simulink model "warplab_mimo_4x4"  (Simulink 6.5)
settings: Solver=ode45  StartTime=0.0  StopTime=20000  RelTol=1e-3
undefined symbols (not defined in the file): gcbh, xlBlockLoadCallback
libraries: xbsIndex_r4 x188
(part 1 of 17)
settings Model: Creator=Melissa.Duarte  LastModifiedBy=melissa.duarte
settings DebuggingCC: MultiTaskDSMMsg=warning  MultiTaskCondExecSysMsg=none
settings RTWCC: IncludeERTFirstTime=on

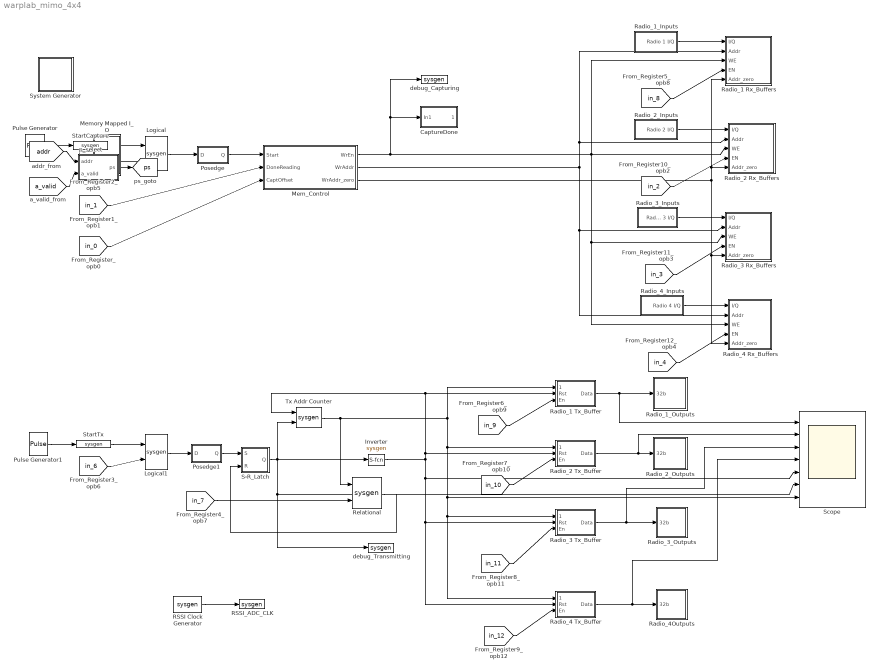
== system warplab_mimo_4x4 ==
  " System Generator" : Subsystem  Tag=genX  mask(Xilinx System Generator Block){infoedit=System Generator, xilinxfamily=virtex2p, part=xc2vp70, speed=-6, package=ff1517, synthesis_tool_sgadvanced=, synthesis_tool=XST, directory=./OPB_Export, testbench_sgadvanced=, testbench=off, simulink_period=1, sysclk_period=10, incr_netlist_sgadvanced=, incr_netlist=off, trim_vbits_sgadvanced=, trim_vbits=Everywhere in SubSystem, dbl_ovrd_sgadvanced=, dbl_ovrd=According to Block Masks, core_generation_sgadvanced=, core_generation=According to Block Masks, run_coregen_sgadvanced=, run_coregen=off, deprecated_control_sgadvanced=, deprecated_control=off, eval_field=0, has_advanced_control=0, sggui_pos=-1,-1,-1,-1, block_type=sysgen, block_version=8.2, sg_icon_stat=51,50,-1,-1,red,beige,0,07734, sg_mask_display=|, sg_list_contents=, sg_blockgui_xml=|}
      mask sg_mask_display=|
      | fprintf('','COMMENT: begin icon graphics');
      | patch([0 51 51 0 ],[0 0 50 50 ],[0.93 0.92 0.86]);
      | patch([12 4 16 4 12 25 29 33 47 36 25 17 29 17 25 36 47 33 29 25 12 ],[5 13 25 37 45 45 41 45 45 34 45 37 25 13 5 16 5 5 9 5 5 ],[0.6 0.2 0.25]);
      | plot([0 0 51 51 0 ],[0 50 50 0 0 ]);
      | fprintf('','COMMENT: end icon graphics');
      | fprintf('','COMMENT: begin icon text');
      | fprintf('','COMMENT: end icon text');
      mask sg_blockgui_xml=|
      | <!--  *  Copyright (c) 2005, Xilinx, Inc.  All Rights Reserved.            --><!--  *  Reproduction or reuse, in any form, without the explicit written  --><!--  *  consent of Xilinx, Inc., is strictly prohibited.                  --><sysgenblock has_userdata="true" tag="genX" block_type="sysgen" simulinkname=" System Generator" >
      |  <icon width="51" bg_color="beige" height="50" caption_format="System\nGenerator" wmark_color="red" />
      |  <callbacks DeleteFcn="xlSysgenGUI('delete', gcs, gcbh);" OpenFcn="xlSysgenGUI('startup',gcs,gcbh)" ModelCloseFcn="xlSysgenGUI('Close',gcs,gcbh)" PostSaveFcn="xlSysgenGUI('Save')" />
      |  <libraries>
      |   <library name="xbsIndex" />
      |   <library name="xbsBasic" />
      |   <library name="xbsTools" />
      |  </libraries>
      |  <subsystem_model file="system_generator_subsystem.mdl" />
      |  <blockgui label="Xilinx System Generator" >
      |   <editbox evaluate="false" multi_line="true" name="infoedit" read_only="true" default=" System Generator" />
      |   <editbox evaluate="false" name="xilinxfamily" default="Virtex4" label="Xilinx family" />
      |   <editbox evaluate="false" name="part" default="xc4vsx35" label="Part" />
      |   <editbox evaluate="false" name="speed" default="-10" label="Speed" />
      |   <editbox evaluate="false" name="package" default="ff668" label="Package" />
      |   <listbox evaluate="true" name="synthesis_tool" default="XST" label="Synthesis tool" >
      |    <item value="Spectrum" />
      |    <item value="Synplify" />
      |    <item value="Synplify Pro" />
      |    <item value="XST" />
      |    <item value="Precision" />
      |   </listbox>
      |   <editbox evaluate="false" name="directory" default="./netlist" label="Target directory" />
      |   <checkbox evaluate="true" name="testbench" default="off" label="Testbench" />
      |   <editbox evaluate="true" name="simulink_period" default="1" label="Simulink period" />
      |   <editbox evaluate="true" name="sysclk_period" default="10" label="System clock period" />
      |   <checkbox evaluate="true" name="incr_netlist" default="off" label="Incremental netlisting" />
      |   <listbox evaluate="true" name="trim_vbits" default="Everywhere in SubSystem" label="Trim valid bits" >
      |    <item value="According to Block Masks" />
      |    <item value="Everywhere in SubSystem" />
      |    <item value="No Where in SubSystem" />
      |   </listbox>
      |   <listbox evaluate="true" name="dbl_ovrd" default="According to Block Masks" label="Override with doubles" >
      |    <item value="According to Block Masks" />
      |    <item value="Everywhere in SubSystem" />
      |    <item value="No Where in SubSystem" />
      |   </listbox>
      |   <listbox evaluate="true" name="core_generation" default="According to Block Masks" label="Generate cores" >
      |    <item value="According to Block Masks" />
      |    <item value="Everywhere Available" />
      |    <item value="Not Needed - Already Generated" />
      |   </listbox>
      |   <checkbox evaluate="true" name="run_coregen" default="off" label="Run CoreGen" />
      |   <checkbox evaluate="true" name="deprecated_control" default="off" label="Show deprecated controls" />
      |   <hiddenvar evaluate="true" name="eval_field" default="0" />
      |  </blockgui>
      | </sysgenblock>
      mask prompts: infoedit ""; xilinxfamily "Xilinx family"; synthesis_tool_sgadvanced ""; synthesis_tool "Synthesis tool"; directory "Target directory"; testbench_sgadvanced ""; simulink_period "Simulink period"; sysclk_period "System clock period"; incr_netlist_sgadvanced ""; incr_netlist "Incremental netlisting"; trim_vbits_sgadvanced ""; trim_vbits "Trim valid bits"; dbl_ovrd_sgadvanced ""; dbl_ovrd "Override with doubles"; core_generation_sgadvanced ""; core_generation "Generate cores"; run_coregen_sgadvanced ""; run_coregen "Run CoreGen"; deprecated_control_sgadvanced ""; deprecated_control "Show deprecated controls"; eval_field ""; has_advanced_control ""; sggui_pos ""; block_type ""; block_version ""; sg_icon_stat ""; sg_mask_display ""; sg_list_contents ""; sg_blockgui_xml ""
      mask help: System Generator
      mask init:
      | try
      |   tmp_gcb = gcb;
      |   tmp_gcbh = gcbh;
      |   xlMungeMaskParams;
      |   serialized_declarations = '{}';
      |   ptable_ = xlblockprep(get_param(tmp_gcb, 'MaskWSVariables'));
      | catch
      |   global dbgsysgen;
      |   if(~isempty(dbgsysgen) && dbgsysgen)
      |     e = regexprep(lasterr, '\n', '\nError: ');
      |     disp(['Error: While running MaskInit code on block ' tmp_gcb ': ' e]);
      |     error(e);
      |   end
      | end
      settings: AttributesFormatString=System\nGenerator  CopyFcn=xlBlockMoveCallback(gcbh);  DeleteFcn=xlSysgenGUI('delete', gcs, gcbh);  ModelCloseFcn=xlSysgenGUI('Close',gcs,gcbh)  PostSaveFcn=xlSysgenGUI('Save')  OpenFcn=xlSysgenGUI('startup',gcs,gcbh)  MoveFcn=xlBlockMoveCallback(gcbh);
      mask Help: eval('xlWeb(xlhtmldoclink('' System Generator''))');
      mask StyleString: edit,edit,edit,edit,edit,edit,popup(Spectrum|Synplify|Synplify Pro|XST|Precision),edit,edit,checkbox,edit,edit,edit,checkbox,edit,popup(According to Block Masks|Everywhere in SubSystem|No Where in SubSystem),edit,popup(According to Block Masks|Everywhere in SubSystem|No Where in SubSystem),edit,popup(According to Block Masks|Everywhere Available|Not Needed - Already Generated),edit,checkbox,edit,checkbox,edit,edit,edit,edit,edit,edit,edit,edit,edit
      mask Display:
      | fprintf('','COMMENT: begin icon graphics');
      | patch([0 51 51 0 ],[0 0 50 50 ],[0.93 0.92 0.86]);
      | patch([12 4 16 4 12 25 29 33 47 36 25 17 29 17 25 36 47 33 29 25 12 ],[5 13 25 37 45 45 41 45 45 34 45 37 25 13 5 16 5 5 9 5 5 ],[0.6 0.2 0.25]);
      | plot([0 0 51 51 0 ],[0 50 50 0 0 ]);
      | fprintf('','COMMENT: end icon graphics');
      | fprintf('','COMMENT: begin icon text');
      | fprintf('','COMMENT: end icon text');
  CaptureDone : Subsystem
  Inverter : S-Function  LoadFcn=xlBlockLoadCallback(gcbh);  FunctionName=sysgen  Parameters=ptable_  mask(Xilinx Inverter Block){infoedit=Bitwise logical negation (one's complement) operator., en_sgadvanced=, en=off, latency=0, dbl_ovrd_sgadvanced=, dbl_ovrd=off, xl_use_area_sgadvanced=, xl_use_area=off, xl_area=[0,0,0,0,0,0,0], has_advanced_control=0, sggui_pos=20,20,356,237, block_type=inv, block_version=8.2, sg_icon_stat=25,18,1,1,white,blue,0,1ab4a85f, sg_mask_display=|, sg_list_contents=, sg_blockgui_xml=}
      mask sg_mask_display=|
      | fprintf('','COMMENT: begin icon graphics');
      | patch([0 25 25 0 ],[0 0 18 18 ],[0.77 0.82 0.91]);
      | patch([8 5 9 5 8 13 14 15 20 16 12 9 13 9 12 16 20 15 14 13 8 ],[2 5 9 13 16 16 15 16 16 12 16 13 9 5 2 6 2 2 3 2 2 ],[0.98 0.96 0.92]);
      | plot([0 0 25 25 0 ],[0 18 18 0 0 ]);
      | fprintf('','COMMENT: end icon graphics');
      | fprintf('','COMMENT: begin icon text');
      | color('black');disp('not');
      | fprintf('','COMMENT: end icon text');
      mask prompts: infoedit ""; en_sgadvanced ""; en "Provide enable port"; dbl_ovrd_sgadvanced ""; dbl_ovrd "Override with doubles"; xl_use_area_sgadvanced ""; xl_use_area "Define FPGA area for resource estimation"; xl_area "FPGA area [slices, FFs, BRAMs, LUTs, IOBs, emb. mults, TBUFs]"; has_advanced_control ""; sggui_pos ""; block_type ""; block_version ""; sg_icon_stat ""; sg_mask_display ""; sg_list_contents ""; sg_blockgui_xml ""
      mask help: Bitwise logical negation (one's complement) operator.
      mask init:
      | try
      |   tmp_gcb = gcb;
      |   tmp_gcbh = gcbh;
      |   xlMungeMaskParams;
      |   block_config = 'sysgen_blockset:Inverter_config';
      |   serialized_declarations = '{''dbl_ovrd''=>''Int'',''en''=>''Int'',''latency''=>''Int''}';
      |   ptable_ = xlblockprep(get_param(tmp_gcb, 'MaskWSVariables'));
      | catch
      |   global dbgsysgen;
      |   if(~isempty(dbgsysgen) && dbgsysgen)
      |     e = regexprep(lasterr, '\n', '\nError: ');
      |     disp(['Error: While running MaskInit code on block ' tmp_gcb ': ' e]);
      |     error(e);
      |   end
      | end
      settings: CopyFcn=xlBlockMoveCallback(gcbh);  DeleteFcn=xlDestroyGui(gcbh);  ModelCloseFcn=xlDestroyGui(gcbh);  PreSaveFcn=xlBlockPreSaveCallback(gcbh);  PostSaveFcn=xlBlockPostSaveCallback(gcbh);  DestroyFcn=xlDestroyGui(gcbh);  OpenFcn=xlOpenGui(gcbh, 'inv_gui.xml', @xlmagicenablement, -1)  CloseFcn=xlDestroyGui(gcbh);  MoveFcn=xlBlockMoveCallback(gcbh);
      mask Help: eval('xlWeb(xlhtmldoclink(''Inverter''))');
      mask Display:
      | fprintf('','COMMENT: begin icon graphics');
      | patch([0 25 25 0 ],[0 0 18 18 ],[0.77 0.82 0.91]);
      | patch([8 5 9 5 8 13 14 15 20 16 12 9 13 9 12 16 20 15 14 13 8 ],[2 5 9 13 16 16 15 16 16 12 16 13 9 5 2 6 2 2 3 2 2 ],[0.98 0.96 0.92]);
      | plot([0 0 25 25 0 ],[0 18 18 0 0 ]);
      | fprintf('','COMMENT: end icon graphics');
      | fprintf('','COMMENT: begin icon text');
      | color('black');disp('not');
      | fprintf('','COMMENT: end icon text');
  Logical : S-Function  LoadFcn=xlBlockLoadCallback(gcbh);  FunctionName=sysgen  Parameters=ptable_  mask(Xilinx Logical Block Block){logical_function_sgadvanced=, logical_function=OR, inputs=2, en_sgadvanced=, en=off, latency=0, precision_sgadvanced=, precision=Full, arith_type_sgadvanced=, arith_type=Unsigned, n_bits=16, bin_pt=0, align_bp_sgadvanced=, align_bp=on, dbl_ovrd_sgadvanced=, dbl_ovrd=off, xl_use_area_sgadvanced=, xl_use_area=off, xl_area=[0,0,0,0,0,0,0], overflow=, quantization=, has_advanced_control=0, sggui_pos=-1,-1,-1,-1, block_type=logical, block_version=8.2, sg_icon_stat=35,55,2,1,white,blue,0,f4a65842, sg_mask_display=|, sg_list_contents=, sg_blockgui_xml=}
      mask sg_mask_display=|
      | fprintf('','COMMENT: begin icon graphics');
      | patch([0 35 35 0 ],[0 0 55 55 ],[0.77 0.82 0.91]);
      | patch([8 2 10 2 8 17 20 23 33 25 18 13 21 13 18 25 33 23 20 17 8 ],[14 20 28 36 42 42 39 42 42 34 41 36 28 20 15 22 14 14 17 14 14 ],[0.98 0.96 0.92]);
      | plot([0 0 35 35 0 ],[0 55 55 0 0 ]);
      | fprintf('','COMMENT: end icon graphics');
      | fprintf('','COMMENT: begin icon text');
      | color('black');disp('\newlineor\newlinez^{-0}','texmode','on');
      | fprintf('','COMMENT: end icon text');
      mask prompts: logical_function_sgadvanced ""; logical_function "Logical function"; inputs "Number of inputs"; en_sgadvanced ""; en "Provide enable port"; precision_sgadvanced ""; arith_type_sgadvanced ""; arith_type "Output Type"; n_bits "Number of bits"; bin_pt "Binary point"; align_bp_sgadvanced ""; align_bp "Align binary point"; dbl_ovrd_sgadvanced ""; dbl_ovrd "Override with doubles"; xl_use_area_sgadvanced ""; xl_use_area "Define FPGA area for resource estimation"; xl_area "FPGA area [slices, FFs, BRAMs, LUTs, IOBs, emb. mults, TBUFs]"; overflow ""; quantization ""; has_advanced_control ""; sggui_pos ""; block_type ""; block_version ""; sg_icon_stat ""; sg_mask_display ""; sg_list_contents ""; sg_blockgui_xml ""
      mask help: Xilinx Logical Block
      mask init:
      | try
      |   tmp_gcb = gcb;
      |   tmp_gcbh = gcbh;
      |   xlMungeMaskParams;
      |   block_config = 'sysgen_blockset:Logical_config';
      |   serialized_declarations = '{''arith_type''=>''Int'',''bin_pt''=>''Int'',''en''=>''Int'',''inputs''=>''Int'',''latency''=>''Int'',''logical_function''=>''Int'',''n_bits''=>''Int'',''precision''=>''Int'',''sim_engine''=>''Int'',''sysgen_root''=>''String''}';
      |   xllogical_init();
      |   ptable_ = xlblockprep(get_param(tmp_gcb, 'MaskWSVariables'));
      | catch
      |   global dbgsysgen;
      |   if(~isempty(dbgsysgen) && dbgsysgen)
      |     e = regexprep(lasterr, '\n', '\nError: ');
      |     disp(['Error: While running MaskInit code on block ' tmp_gcb ': ' e]);
      |     error(e);
      |   end
      | end
      settings: CopyFcn=xlBlockMoveCallback(gcbh);  DeleteFcn=xlDestroyGui(gcbh);  ModelCloseFcn=xlDestroyGui(gcbh);  PreSaveFcn=xlBlockPreSaveCallback(gcbh);  PostSaveFcn=xlBlockPostSaveCallback(gcbh);  DestroyFcn=xlDestroyGui(gcbh);  OpenFcn=xlOpenGui(gcbh, 'logical_gui.xml', @logicalenablement, -1)  CloseFcn=xlDestroyGui(gcbh);  MoveFcn=xlBlockMoveCallback(gcbh);
      mask Help: eval('xlWeb(xlhtmldoclink(''Logical''))');
      mask StyleString: edit,popup(AND|NAND|OR|NOR|XOR|XNOR),edit,edit,checkbox,edit,edit,popup(Full|User Defined),edit,popup(Signed  (2's comp)|Unsigned),edit,edit,edit,checkbox,edit,checkbox,edit,checkbox,edit,edit,edit,edit,edit,edit,edit,edit,edit,edit,edit
      mask Display:
      | fprintf('','COMMENT: begin icon graphics');
      | patch([0 35 35 0 ],[0 0 55 55 ],[0.77 0.82 0.91]);
      | patch([8 2 10 2 8 17 20 23 33 25 18 13 21 13 18 25 33 23 20 17 8 ],[14 20 28 36 42 42 39 42 42 34 41 36 28 20 15 22 14 14 17 14 14 ],[0.98 0.96 0.92]);
      | plot([0 0 35 35 0 ],[0 55 55 0 0 ]);
      | fprintf('','COMMENT: end icon graphics');
      | fprintf('','COMMENT: begin icon text');
      | color('black');disp('\newlineor\newlinez^{-0}','texmode','on');
      | fprintf('','COMMENT: end icon text');
  Logical1 : S-Function  LoadFcn=xlBlockLoadCallback(gcbh);  FunctionName=sysgen  Parameters=ptable_  mask(Xilinx Logical Block Block){logical_function_sgadvanced=, logical_function=OR, inputs=2, en_sgadvanced=, en=off, latency=0, precision_sgadvanced=, precision=Full, arith_type_sgadvanced=, arith_type=Unsigned, n_bits=16, bin_pt=0, align_bp_sgadvanced=, align_bp=on, dbl_ovrd_sgadvanced=, dbl_ovrd=off, xl_use_area_sgadvanced=, xl_use_area=off, xl_area=[0,0,0,0,0,0,0], overflow=, quantization=, has_advanced_control=0, sggui_pos=-1,-1,-1,-1, block_type=logical, block_version=8.2, sg_icon_stat=35,55,2,1,white,blue,0,f4a65842, sg_mask_display=|, sg_list_contents=, sg_blockgui_xml=}
      mask sg_mask_display=|
      | fprintf('','COMMENT: begin icon graphics');
      | patch([0 35 35 0 ],[0 0 55 55 ],[0.77 0.82 0.91]);
      | patch([8 2 10 2 8 17 20 23 33 25 18 13 21 13 18 25 33 23 20 17 8 ],[14 20 28 36 42 42 39 42 42 34 41 36 28 20 15 22 14 14 17 14 14 ],[0.98 0.96 0.92]);
      | plot([0 0 35 35 0 ],[0 55 55 0 0 ]);
      | fprintf('','COMMENT: end icon graphics');
      | fprintf('','COMMENT: begin icon text');
      | color('black');disp('\newlineor\newlinez^{-0}','texmode','on');
      | fprintf('','COMMENT: end icon text');
      mask prompts: logical_function_sgadvanced ""; logical_function "Logical function"; inputs "Number of inputs"; en_sgadvanced ""; en "Provide enable port"; precision_sgadvanced ""; arith_type_sgadvanced ""; arith_type "Output Type"; n_bits "Number of bits"; bin_pt "Binary point"; align_bp_sgadvanced ""; align_bp "Align binary point"; dbl_ovrd_sgadvanced ""; dbl_ovrd "Override with doubles"; xl_use_area_sgadvanced ""; xl_use_area "Define FPGA area for resource estimation"; xl_area "FPGA area [slices, FFs, BRAMs, LUTs, IOBs, emb. mults, TBUFs]"; overflow ""; quantization ""; has_advanced_control ""; sggui_pos ""; block_type ""; block_version ""; sg_icon_stat ""; sg_mask_display ""; sg_list_contents ""; sg_blockgui_xml ""
      mask help: Xilinx Logical Block
      mask init: same as warplab_mimo_4x4/Logical
      settings: CopyFcn=xlBlockMoveCallback(gcbh);  DeleteFcn=xlDestroyGui(gcbh);  ModelCloseFcn=xlDestroyGui(gcbh);  PreSaveFcn=xlBlockPreSaveCallback(gcbh);  PostSaveFcn=xlBlockPostSaveCallback(gcbh);  DestroyFcn=xlDestroyGui(gcbh);  OpenFcn=xlOpenGui(gcbh, 'logical_gui.xml', @logicalenablement, -1)  CloseFcn=xlDestroyGui(gcbh);  MoveFcn=xlBlockMoveCallback(gcbh);
      mask Help: eval('xlWeb(xlhtmldoclink(''Logical''))');
      mask StyleString: edit,popup(AND|NAND|OR|NOR|XOR|XNOR),edit,edit,checkbox,edit,edit,popup(Full|User Defined),edit,popup(Signed  (2's comp)|Unsigned),edit,edit,edit,checkbox,edit,checkbox,edit,checkbox,edit,edit,edit,edit,edit,edit,edit,edit,edit,edit,edit
      mask Display:
      | fprintf('','COMMENT: begin icon graphics');
      | patch([0 35 35 0 ],[0 0 55 55 ],[0.77 0.82 0.91]);
      | patch([8 2 10 2 8 17 20 23 33 25 18 13 21 13 18 25 33 23 20 17 8 ],[14 20 28 36 42 42 39 42 42 34 41 36 28 20 15 22 14 14 17 14 14 ],[0.98 0.96 0.92]);
      | plot([0 0 35 35 0 ],[0 55 55 0 0 ]);
      | fprintf('','COMMENT: end icon graphics');
      | fprintf('','COMMENT: begin icon text');
      | color('black');disp('\newlineor\newlinez^{-0}','texmode','on');
      | fprintf('','COMMENT: end icon text');
  Mem_Control : Subsystem
  Memory Mapped I_O : Subsystem
  Posedge : Subsystem
  Posedge1 : Subsystem
  Pulse Generator : DiscretePulseGenerator  Period=1000000  PulseWidth=50  PhaseDelay=2
  Pulse Generator1 : DiscretePulseGenerator  Period=1000000  PulseWidth=50  PhaseDelay=2
  RSSI Clock Generator : S-Function  LoadFcn=xlBlockLoadCallback(gcbh);  FunctionName=sysgen  Parameters=ptable_  mask(Xilinx Counter Block){infoedit=Hardware notes: Free running counters are the least expensive in hardware.  A count limited counter is implemented by combining a counter with a comparator., cnt_type_sgadvanced=, cnt_type=Free Running, cnt_to=Inf, operation_sgadvanced=, operation=Up, start_count=0, cnt_by_val=1, arith_type_sgadvanced=, arith_type=Unsigned, n_bits=1, bin_pt=0, load_pin_sgadvanced=, load_pin=off, rst_sgadvanced=, rst=off, en_sgadvanced=, en=off, explicit_period_sgadvanced=, explicit_period=on, period=2, dbl_ovrd_sgadvanced=, dbl_ovrd=off, use_behavioral_HDL_sgadvanced=, use_behavioral_HDL=off, use_rpm_sgadvanced=, use_rpm=off, xl_use_area_sgadvanced=, xl_use_area=off, xl_area=[0,0,0,0,0,0,0], xlcconfig=, has_advanced_control=0, sggui_pos=20,20,356,630, block_type=counter, block_version=VER_STRING_GOES_HERE, sg_icon_stat=45,26,0,1,white,blue,0,115399eb, sg_mask_display=|, sg_list_contents=, sg_blockgui_xml=}
      mask sg_mask_display=|
      | fprintf('','COMMENT: begin icon graphics ');
      | patch([0 45 45 0 ],[0 0 26 26 ],[0.77 0.82 0.91]);
      | patch([15 11 17 11 15 22 24 26 33 27 21 17 23 17 21 27 33 26 24 22 15 ],[3 7 13 19 23 23 21 23 23 17 23 19 13 7 3 9 3 3 5 3 3 ],[0.98 0.96 0.92]);
      | plot([0 0 45 45 0 ],[0 26 26 0 0 ]);
      | fprintf('','COMMENT: end icon graphics');
      |
      | fprintf('','COMMENT: begin icon text ');
      | color('black');port_label('output',1,'out');
      | fprintf('','COMMENT: end icon text');
      mask prompts: infoedit ""; cnt_type_sgadvanced ""; cnt_type "Counter type"; cnt_to "Count to value"; operation_sgadvanced ""; operation "Count direction"; start_count "Initial value"; cnt_by_val "Step"; arith_type_sgadvanced ""; arith_type "Output type"; n_bits "Number of bits"; bin_pt "Binary point"; load_pin_sgadvanced ""; load_pin "Provide load port"; rst_sgadvanced ""; rst "Provide synchronous reset port"; en_sgadvanced ""; en "Provide enable port"; explicit_period_sgadvanced ""; explicit_period "Sample period source"; period "Explicit period"; dbl_ovrd_sgadvanced ""; dbl_ovrd "Override with doubles"; use_behavioral_HDL_sgadvanced ""; use_behavioral_HDL "Use behavioral HDL (otherwise use core)"; use_rpm_sgadvanced ""; use_rpm "Use pre-defined core placement information"; xl_use_area_sgadvanced ""; xl_use_area "Define FPGA area for resource estimation"; xl_area "FPGA area [slices, FFs, BRAMs, LUTs, IOBs, emb. mults, TBUFs]"; xlcconfig ""; has_advanced_control ""; sggui_pos ""; block_type ""; block_version ""; sg_icon_stat ""; sg_mask_display ""; sg_list_contents ""; sg_blockgui_xml ""
      mask help: Hardware notes: Free running counters are the least expensive in hardware. A count limited counter is implemented by combining a counter with a comparator.
      mask init:
      | try
      |   tmp_gcb = gcb;
      |   tmp_gcbh = gcbh;
      |   xlMungeMaskParams;
      |   block_config = 'sysgen_blockset:Counter_config';
      |   serialized_declarations = '{''arith_type''=>''Int'',''bin_pt''=>''Int'',''cnt_by_val''=>''Double'',''cnt_to''=>''Double'',''cnt_type''=>''Int'',''en''=>''Int'',''explicit_period''=>''Int'',''load_pin''=>''Int'',''n_bits''=>''Int'',''operation''=>''Int'',''period''=>''Double'',''rst''=>''Int'',''start_count''=>''Double'',''use_behavioral_HDL''=>''Int'',''use_rpm''=>''Int'',''xlcconfig''=>''String''}';
      |   ptable_ = xlblockprep(get_param(tmp_gcb, 'MaskWSVariables'));
      | catch
      |   global dbgsysgen;
      |   if(~isempty(dbgsysgen) && dbgsysgen)
      |     e = regexprep(lasterr, '\n', '\nError: ');
      |     disp(['Error: While running MaskInit code on block ' tmp_gcb ': ' e]);
      |     error(e);
      |   end
      | end
      settings: CopyFcn=xlBlockMoveCallback(gcbh);  DeleteFcn=xlDestroyGui(gcbh);  ModelCloseFcn=xlDestroyGui(gcbh);  PreSaveFcn=xlBlockPreSaveCallback(gcbh);  PostSaveFcn=xlBlockPostSaveCallback(gcbh);  DestroyFcn=xlDestroyGui(gcbh);  OpenFcn=xlOpenGui(gcbh, 'counter_gui.xml', @counterenablement, -1)  CloseFcn=xlDestroyGui(gcbh);  MoveFcn=xlBlockMoveCallback(gcbh);
      mask Help: eval('xlWeb(xlhtmldoclink(''Counter''))');
      mask StyleString: edit,edit,popup(Free Running|Count Limited),edit,edit,popup(Up|Down|Up/Down),edit,edit,edit,popup(Signed  (2's comp)|Unsigned),edit,edit,edit,checkbox,edit,checkbox,edit,checkbox,edit,popup(on|off),edit,edit,checkbox,edit,checkbox,edit,checkbox,edit,checkbox,edit,edit,edit,edit,edit,edit,edit,edit,edit,edit
      mask Display:
      | fprintf('','COMMENT: begin icon graphics ');
      | patch([0 45 45 0 ],[0 0 26 26 ],[0.77 0.82 0.91]);
      | patch([15 11 17 11 15 22 24 26 33 27 21 17 23 17 21 27 33 26 24 22 15 ],[3 7 13 19 23 23 21 23 23 17 23 19 13 7 3 9 3 3 5 3 3 ],[0.98 0.96 0.92]);
      | plot([0 0 45 45 0 ],[0 26 26 0 0 ]);
      | fprintf('','COMMENT: end icon graphics');
      | 
      | fprintf('','COMMENT: begin icon text ');
      | color('black');port_label('output',1,'out');
      | fprintf('','COMMENT: end icon text');
  RSSI_ADC_CLK : S-Function  LoadFcn=xlBlockLoadCallback(gcbh);  FunctionName=sysgen  Parameters=ptable_  mask(Xilinx Gateway Out Block){infoedit=Gateway out block.  Converts Xilinx fixed point inputs into ouputs of type Simulink integer, double, or fixed point.<P><P>Hardware notes:  In hardware these blocks become top level output ports or are discarded, depending on how they are configured., hdl_port_sgadvanced=, hdl_port=on, timing_constraint_sgadvanced=, timing_constraint=None, locs_specified_sgadvanced=, locs_specified=off, LOCs={}, xl_use_area_sgadvanced=, xl_use_area=off, xl_area=[0,0,0,0,0,0,0], sginterface=, has_advanced_control=0, sggui_pos=-1,-1,-1,-1, block_type=gatewayout, block_version=8.2, sg_icon_stat=40,14,1,1,white,yellow,0,f0cec300, sg_mask_display=|, sg_list_contents=, sg_blockgui_xml=}
      mask sg_mask_display=|
      | fprintf('','COMMENT: begin icon graphics');
      | patch([0 40 40 0 ],[0 0 14 14 ],[0.95 0.93 0.65]);
      | patch([16 14 17 14 16 20 21 22 26 23 20 18 21 18 20 23 26 22 21 20 16 ],[2 4 7 10 12 12 11 12 12 9 12 10 7 4 2 5 2 2 3 2 2 ],[0.98 0.96 0.92]);
      | plot([0 0 40 40 0 ],[0 14 14 0 0 ]);
      | fprintf('','COMMENT: end icon graphics');
      | fprintf('','COMMENT: begin icon text');
      | color('black');port_label('input',1,' ');
      | color('black');port_label('output',1,'\fontsize{11pt}\bf Out ','texmode','on');
      | fprintf('','COMMENT: end icon text');
      mask prompts: infoedit ""; hdl_port_sgadvanced ""; hdl_port "Translate into output port"; timing_constraint_sgadvanced ""; timing_constraint "IOB timing constraint"; locs_specified_sgadvanced ""; locs_specified "Specify IOB location constraints"; LOCs "IOB pad locations (cell array {'MSB', ..., 'LSB'})"; xl_use_area_sgadvanced ""; xl_use_area "Define FPGA area for resource estimation"; xl_area "FPGA area [slices, FFs, BRAMs, LUTs, IOBs, emb. mults, TBUFs]"; sginterface ""; has_advanced_control ""; sggui_pos ""; block_type ""; block_version ""; sg_icon_stat ""; sg_mask_display ""; sg_list_contents ""; sg_blockgui_xml ""
      mask help:
      | Gateway out block.  Converts Xilinx fixed point inputs into ouputs of type Simulink integer, double, or fixed point.
      |
      | Hardware notes:  In hardware these blocks become top level output ports or are discarded, depending on how they are configured.
      mask init:
      | try
      |   tmp_gcb = gcb;
      |   tmp_gcbh = gcbh;
      |   xlMungeMaskParams;
      |   block_config = 'sysgen_blockset:gateway_out_config';
      |   serialized_declarations = '{''LOCs''=>''StringVector'',''hdl_port''=>''Int'',''locs_specified''=>''Int'',''sginterface''=>''String'',''timing_constraint''=>''Int''}';
      |   ptable_ = xlblockprep(get_param(tmp_gcb, 'MaskWSVariables'));
      | catch
      |   global dbgsysgen;
      |   if(~isempty(dbgsysgen) && dbgsysgen)
      |     e = regexprep(lasterr, '\n', '\nError: ');
      |     disp(['Error: While running MaskInit code on block ' tmp_gcb ': ' e]);
      |     error(e);
      |   end
      | end
      settings: CopyFcn=xlBlockMoveCallback(gcbh);  DeleteFcn=xlDestroyGui(gcbh);  ModelCloseFcn=xlDestroyGui(gcbh);  PreSaveFcn=xlBlockPreSaveCallback(gcbh);  PostSaveFcn=xlBlockPostSaveCallback(gcbh);  DestroyFcn=xlDestroyGui(gcbh);  OpenFcn=xlOpenGui(gcbh, 'gatewayout_gui.xml', @gatewayoutenablement, -1)  CloseFcn=xlDestroyGui(gcbh);  MoveFcn=xlBlockMoveCallback(gcbh);
      mask Help: eval('xlWeb(xlhtmldoclink(''Gateway Out''))');
      mask StyleString: edit,edit,checkbox,edit,popup(None|Data Rate|Data Rate;  Set 'FAST' Attribute),edit,checkbox,edit,edit,checkbox,edit,edit,edit,edit,edit,edit,edit,edit,edit,edit
      mask Display:
      | fprintf('','COMMENT: begin icon graphics');
      | patch([0 40 40 0 ],[0 0 14 14 ],[0.95 0.93 0.65]);
      | patch([16 14 17 14 16 20 21 22 26 23 20 18 21 18 20 23 26 22 21 20 16 ],[2 4 7 10 12 12 11 12 12 9 12 10 7 4 2 5 2 2 3 2 2 ],[0.98 0.96 0.92]);
      | plot([0 0 40 40 0 ],[0 14 14 0 0 ]);
      | fprintf('','COMMENT: end icon graphics');
      | fprintf('','COMMENT: begin icon text');
      | color('black');port_label('input',1,' ');
      | color('black');port_label('output',1,'\fontsize{11pt}\bf Out ','texmode','on');
      | fprintf('','COMMENT: end icon text');
  Radio_1 Rx_Buffers : Subsystem
  Radio_1 Tx_Buffer : Subsystem
  Radio_1_Inputs : Subsystem
  Radio_1_Outputs : Subsystem
  Radio_2 Rx_Buffers : Subsystem
  Radio_2 Tx_Buffer : Subsystem
  Radio_2_Inputs : Subsystem
  Radio_2_Outputs : Subsystem
  Radio_3 Rx_Buffers : Subsystem
  Radio_3 Tx_Buffer : Subsystem
  Radio_3_Inputs : Subsystem
  Radio_3_Outputs : Subsystem
  Radio_4 Rx_Buffers : Subsystem
  Radio_4 Tx_Buffer : Subsystem
  Radio_4Outputs : Subsystem
  Radio_4_Inputs : Subsystem
  Relational : S-Function  LoadFcn=xlBlockLoadCallback(gcbh);  FunctionName=sysgen  Parameters=ptable_  mask(Xilinx Arithmetic Relational Operator Block){mode_sgadvanced=, mode=a>=b, en_sgadvanced=, en=off, latency=0, dbl_ovrd_sgadvanced=, dbl_ovrd=off, xl_use_area_sgadvanced=, xl_use_area=off, xl_area=[0,0,0,0,0,0,0], has_advanced_control=0, sggui_pos=-1,-1,-1,-1, block_type=relational, block_version=8.2, sg_icon_stat=45,49,2,1,white,blue,0,6d6ac162, sg_mask_display=|, sg_list_contents=, sg_blockgui_xml=}
      mask sg_mask_display=|
      | fprintf('','COMMENT: begin icon graphics');
      | patch([0 45 45 0 ],[0 0 49 49 ],[0.77 0.82 0.91]);
      | patch([10 3 14 3 10 22 25 28 41 31 21 14 25 14 21 31 41 28 25 22 10 ],[7 14 25 36 43 43 40 43 43 33 43 36 25 14 7 17 7 7 10 7 7 ],[0.98 0.96 0.92]);
      | plot([0 0 45 45 0 ],[0 49 49 0 0 ]);
      | fprintf('','COMMENT: end icon graphics');
      | fprintf('','COMMENT: begin icon text');
      | color('black');port_label('input',1,'a');
      | color('black');port_label('input',2,'b');
      | color('black');disp('\newline\bf{a>=b}\newlinez^{-0}','texmode','on');
      | fprintf('','COMMENT: end icon text');
      mask prompts: mode_sgadvanced ""; mode "Comparison:"; en_sgadvanced ""; en "Provide enable port"; dbl_ovrd_sgadvanced ""; dbl_ovrd "Override with doubles"; xl_use_area_sgadvanced ""; xl_use_area "Define FPGA area for resource estimation"; xl_area "FPGA area [slices, FFs, BRAMs, LUTs, IOBs, emb. mults, TBUFs]"; has_advanced_control ""; sggui_pos ""; block_type ""; block_version ""; sg_icon_stat ""; sg_mask_display ""; sg_list_contents ""; sg_blockgui_xml ""
      mask help: Xilinx Arithmetic Relational Operator
      mask init:
      | try
      |   tmp_gcb = gcb;
      |   tmp_gcbh = gcbh;
      |   xlMungeMaskParams;
      |   block_config = 'sysgen_blockset:Relational_config';
      |   serialized_declarations = '{''dbl_ovrd''=>''Int'',''en''=>''Int'',''latency''=>''Int'',''mode''=>''Int''}';
      |   ptable_ = xlblockprep(get_param(tmp_gcb, 'MaskWSVariables'));
      | catch
      |   global dbgsysgen;
      |   if(~isempty(dbgsysgen) && dbgsysgen)
      |     e = regexprep(lasterr, '\n', '\nError: ');
      |     disp(['Error: While running MaskInit code on block ' tmp_gcb ': ' e]);
      |     error(e);
      |   end
      | end
      settings: CopyFcn=xlBlockMoveCallback(gcbh);  DeleteFcn=xlDestroyGui(gcbh);  ModelCloseFcn=xlDestroyGui(gcbh);  PreSaveFcn=xlBlockPreSaveCallback(gcbh);  PostSaveFcn=xlBlockPostSaveCallback(gcbh);  DestroyFcn=xlDestroyGui(gcbh);  OpenFcn=xlOpenGui(gcbh, 'relational_gui.xml', @xlmagicenablement, -1)  CloseFcn=xlDestroyGui(gcbh);  MoveFcn=xlBlockMoveCallback(gcbh);
      mask Help: eval('xlWeb(xlhtmldoclink(''Relational''))');
      mask StyleString: edit,popup(a=b|a!=b|a<b|a>b|a<=b|a>=b),edit,checkbox,edit,edit,checkbox,edit,checkbox,edit,edit,edit,edit,edit,edit,edit,edit,edit
      mask Display:
      | fprintf('','COMMENT: begin icon graphics');
      | patch([0 45 45 0 ],[0 0 49 49 ],[0.77 0.82 0.91]);
      | patch([10 3 14 3 10 22 25 28 41 31 21 14 25 14 21 31 41 28 25 22 10 ],[7 14 25 36 43 43 40 43 43 33 43 36 25 14 7 17 7 7 10 7 7 ],[0.98 0.96 0.92]);
      | plot([0 0 45 45 0 ],[0 49 49 0 0 ]);
      | fprintf('','COMMENT: end icon graphics');
      | fprintf('','COMMENT: begin icon text');
      | color('black');port_label('input',1,'a');
      | color('black');port_label('input',2,'b');
      | color('black');disp('\newline\bf{a>=b}\newlinez^{-0}','texmode','on');
      | fprintf('','COMMENT: end icon text');
  S-R_Latch : Subsystem
  Scope : Scope  NumInputPorts=7
      settings: YMin=-5~-5~-5~-5~-5~-5~-5  YMax=5~5~5~5~5~5~5  SaveName=ScopeData2  MaxDataPoints=50000
  StartCapture : S-Function  LoadFcn=xlBlockLoadCallback(gcbh);  FunctionName=sysgen  Parameters=ptable_  mask(Xilinx Gateway In Block){infoedit=Gateway in block.  Converts inputs of type Simulink integer, double and fixed point to  Xilinx fixed point type.<P><P>Hardware notes:  In hardware these blocks become top level input ports., arith_type_sgadvanced=, arith_type=Unsigned, n_bits=1, bin_pt=0, quantization_sgadvanced=, quantization=Round  (unbiased: +/- Inf), overflow_sgadvanced=, overflow=Saturate, period=1, dbl_ovrd_sgadvanced=, dbl_ovrd=off, timing_constraint_sgadvanced=, timing_constraint=None, locs_specified_sgadvanced=, locs_specified=off, LOCs={}, xl_use_area_sgadvanced=, xl_use_area=off, xl_area=[0,0,0,0,0,0,0], sginterface=, has_advanced_control=0, sggui_pos=20,20,356,432, block_type=gatewayin, block_version=VER_STRING_GOES_HERE, sg_icon_stat=55,12,1,1,white,yellow,0,4bb76ffd, sg_mask_display=|, sg_list_contents=, sg_blockgui_xml=}
      mask sg_mask_display=|
      | fprintf('','COMMENT: begin icon graphics ');
      | patch([0 55 55 0 ],[0 0 12 12 ],[0.95 0.93 0.65]);
      | patch([24 22 25 22 24 27 28 29 32 29 26 24 27 24 26 29 32 29 28 27 24 ],[1 3 6 9 11 11 10 11 11 8 11 9 6 3 1 4 1 1 2 1 1 ],[0.98 0.96 0.92]);
      | plot([0 0 55 55 0 ],[0 12 12 0 0 ]);
      | fprintf('','COMMENT: end icon graphics');
      |
      | fprintf('','COMMENT: begin icon text ');
      | color('black');port_label('input',1,'\fontsize{11pt}\bf In ','texmode','on');
      | color('black');port_label('output',1,' ');
      | fprintf('','COMMENT: end icon text');
      | fprintf('','COMMENT: Make no changes above this line -- machine generated code. ');
      mask prompts: infoedit ""; arith_type_sgadvanced ""; arith_type "Output type"; n_bits "Number of bits"; bin_pt "Binary point"; quantization_sgadvanced ""; overflow_sgadvanced ""; period "Sample period"; dbl_ovrd_sgadvanced ""; dbl_ovrd "Override with doubles"; timing_constraint_sgadvanced ""; timing_constraint "IOB timing constraint"; locs_specified_sgadvanced ""; locs_specified "Specify IOB location constraints"; LOCs "IOB pad locations (specify as cell array {'MSB', ..., 'LSB'})"; xl_use_area_sgadvanced ""; xl_use_area "Define FPGA area for resource estimation"; xl_area "FPGA area [slices, FFs, BRAMs, LUTs, IOBs, emb. mults, TBUFs]"; sginterface ""; has_advanced_control ""; sggui_pos ""; block_type ""; block_version ""; sg_icon_stat ""; sg_mask_display ""; sg_list_contents ""; sg_blockgui_xml ""
      mask help:
      | Gateway in block.  Converts inputs of type Simulink integer, double and fixed point to  Xilinx fixed point type.
      |
      | Hardware notes:  In hardware these blocks become top level input ports.
      mask init:
      | try
      |   tmp_gcb = gcb;
      |   tmp_gcbh = gcbh;
      |   xlMungeMaskParams;
      |   block_config = 'sysgen_blockset:gateway_in_config';
      |   serialized_declarations = '{''LOCs''=>''StringVector'',''arith_type''=>''Int'',''bin_pt''=>''Int'',''locs_specified''=>''Int'',''n_bits''=>''Int'',''overflow''=>''Int'',''period''=>''Double'',''quantization''=>''Int'',''sginterface''=>''String'',''timing_constraint''=>''Int''}';
      |   ptable_ = xlblockprep(get_param(tmp_gcb, 'MaskWSVariables'));
      | catch
      |   global dbgsysgen;
      |   if(~isempty(dbgsysgen) && dbgsysgen)
      |     e = regexprep(lasterr, '\n', '\nError: ');
      |     disp(['Error: While running MaskInit code on block ' tmp_gcb ': ' e]);
      |     error(e);
      |   end
      | end
      settings: CopyFcn=xlBlockMoveCallback(gcbh);  DeleteFcn=xlDestroyGui(gcbh);  ModelCloseFcn=xlDestroyGui(gcbh);  PreSaveFcn=xlBlockPreSaveCallback(gcbh);  PostSaveFcn=xlBlockPostSaveCallback(gcbh);  DestroyFcn=xlDestroyGui(gcbh);  OpenFcn=xlOpenGui(gcbh, 'gatewayin_gui.xml', @gatewayinenablement, @gatewayinaction)  CloseFcn=xlDestroyGui(gcbh);  MoveFcn=xlBlockMoveCallback(gcbh);
      mask Help: eval('xlWeb(xlhtmldoclink(''Gateway In''))');
      mask StyleString: edit,edit,popup(Boolean|Signed  (2's comp)|Unsigned),edit,edit,edit,popup(Truncate|Round  (unbiased: +/- Inf)),edit,popup(Wrap|Saturate|Flag as error),edit,edit,checkbox,edit,popup(None|Data Rate),edit,checkbox,edit,edit,checkbox,edit,edit,edit,edit,edit,edit,edit,edit,edit,edit
      mask Display:
      | fprintf('','COMMENT: begin icon graphics ');
      | patch([0 55 55 0 ],[0 0 12 12 ],[0.95 0.93 0.65]);
      | patch([24 22 25 22 24 27 28 29 32 29 26 24 27 24 26 29 32 29 28 27 24 ],[1 3 6 9 11 11 10 11 11 8 11 9 6 3 1 4 1 1 2 1 1 ],[0.98 0.96 0.92]);
      | plot([0 0 55 55 0 ],[0 12 12 0 0 ]);
      | fprintf('','COMMENT: end icon graphics');
      | 
      | fprintf('','COMMENT: begin icon text ');
      | color('black');port_label('input',1,'\fontsize{11pt}\bf In ','texmode','on');
      | color('black');port_label('output',1,' ');
      | fprintf('','COMMENT: end icon text');
      | fprintf('','COMMENT: Make no changes above this line -- machine generated code. ');
  StartTx : S-Function  LoadFcn=xlBlockLoadCallback(gcbh);  FunctionName=sysgen  Parameters=ptable_  mask(Xilinx Gateway In Block){infoedit=Gateway in block.  Converts inputs of type Simulink integer, double and fixed point to  Xilinx fixed point type.<P><P>Hardware notes:  In hardware these blocks become top level input ports., arith_type_sgadvanced=, arith_type=Unsigned, n_bits=1, bin_pt=0, quantization_sgadvanced=, quantization=Round  (unbiased: +/- Inf), overflow_sgadvanced=, overflow=Saturate, period=1, dbl_ovrd_sgadvanced=, dbl_ovrd=off, timing_constraint_sgadvanced=, timing_constraint=None, locs_specified_sgadvanced=, locs_specified=off, LOCs={}, xl_use_area_sgadvanced=, xl_use_area=off, xl_area=[0,0,0,0,0,0,0], sginterface=, has_advanced_control=0, sggui_pos=20,20,356,432, block_type=gatewayin, block_version=VER_STRING_GOES_HERE, sg_icon_stat=55,12,1,1,white,yellow,0,4bb76ffd, sg_mask_display=|, sg_list_contents=, sg_blockgui_xml=}
      mask sg_mask_display=|
      | fprintf('','COMMENT: begin icon graphics ');
      | patch([0 55 55 0 ],[0 0 12 12 ],[0.95 0.93 0.65]);
      | patch([24 22 25 22 24 27 28 29 32 29 26 24 27 24 26 29 32 29 28 27 24 ],[1 3 6 9 11 11 10 11 11 8 11 9 6 3 1 4 1 1 2 1 1 ],[0.98 0.96 0.92]);
      | plot([0 0 55 55 0 ],[0 12 12 0 0 ]);
      | fprintf('','COMMENT: end icon graphics');
      |
      | fprintf('','COMMENT: begin icon text ');
      | color('black');port_label('input',1,'\fontsize{11pt}\bf In ','texmode','on');
      | color('black');port_label('output',1,' ');
      | fprintf('','COMMENT: end icon text');
      | fprintf('','COMMENT: Make no changes above this line -- machine generated code. ');
      mask prompts: infoedit ""; arith_type_sgadvanced ""; arith_type "Output type"; n_bits "Number of bits"; bin_pt "Binary point"; quantization_sgadvanced ""; overflow_sgadvanced ""; period "Sample period"; dbl_ovrd_sgadvanced ""; dbl_ovrd "Override with doubles"; timing_constraint_sgadvanced ""; timing_constraint "IOB timing constraint"; locs_specified_sgadvanced ""; locs_specified "Specify IOB location constraints"; LOCs "IOB pad locations (specify as cell array {'MSB', ..., 'LSB'})"; xl_use_area_sgadvanced ""; xl_use_area "Define FPGA area for resource estimation"; xl_area "FPGA area [slices, FFs, BRAMs, LUTs, IOBs, emb. mults, TBUFs]"; sginterface ""; has_advanced_control ""; sggui_pos ""; block_type ""; block_version ""; sg_icon_stat ""; sg_mask_display ""; sg_list_contents ""; sg_blockgui_xml ""
      mask help:
      | Gateway in block.  Converts inputs of type Simulink integer, double and fixed point to  Xilinx fixed point type.
      |
      | Hardware notes:  In hardware these blocks become top level input ports.
      mask init: same as warplab_mimo_4x4/StartCapture
      settings: CopyFcn=xlBlockMoveCallback(gcbh);  DeleteFcn=xlDestroyGui(gcbh);  ModelCloseFcn=xlDestroyGui(gcbh);  PreSaveFcn=xlBlockPreSaveCallback(gcbh);  PostSaveFcn=xlBlockPostSaveCallback(gcbh);  DestroyFcn=xlDestroyGui(gcbh);  OpenFcn=xlOpenGui(gcbh, 'gatewayin_gui.xml', @gatewayinenablement, @gatewayinaction)  CloseFcn=xlDestroyGui(gcbh);  MoveFcn=xlBlockMoveCallback(gcbh);
      mask Help: eval('xlWeb(xlhtmldoclink(''Gateway In''))');
      mask StyleString: edit,edit,popup(Boolean|Signed  (2's comp)|Unsigned),edit,edit,edit,popup(Truncate|Round  (unbiased: +/- Inf)),edit,popup(Wrap|Saturate|Flag as error),edit,edit,checkbox,edit,popup(None|Data Rate),edit,checkbox,edit,edit,checkbox,edit,edit,edit,edit,edit,edit,edit,edit,edit,edit
      mask Display:
      | fprintf('','COMMENT: begin icon graphics ');
      | patch([0 55 55 0 ],[0 0 12 12 ],[0.95 0.93 0.65]);
      | patch([24 22 25 22 24 27 28 29 32 29 26 24 27 24 26 29 32 29 28 27 24 ],[1 3 6 9 11 11 10 11 11 8 11 9 6 3 1 4 1 1 2 1 1 ],[0.98 0.96 0.92]);
      | plot([0 0 55 55 0 ],[0 12 12 0 0 ]);
      | fprintf('','COMMENT: end icon graphics');
      | 
      | fprintf('','COMMENT: begin icon text ');
      | color('black');port_label('input',1,'\fontsize{11pt}\bf In ','texmode','on');
      | color('black');port_label('output',1,' ');
      | fprintf('','COMMENT: end icon text');
      | fprintf('','COMMENT: Make no changes above this line -- machine generated code. ');
  Tx Addr Counter : S-Function  LoadFcn=xlBlockLoadCallback(gcbh);  FunctionName=sysgen  Parameters=ptable_  mask(Xilinx Counter Block){infoedit=Hardware notes: Free running counters are the least expensive in hardware.  A count limited counter is implemented by combining a counter with a comparator., cnt_type_sgadvanced=, cnt_type=Free Running, cnt_to=Inf, operation_sgadvanced=, operation=Up, start_count=0, cnt_by_val=1, arith_type_sgadvanced=, arith_type=Unsigned, n_bits=14, bin_pt=0, load_pin_sgadvanced=, load_pin=off, rst_sgadvanced=, rst=on, en_sgadvanced=, en=on, explicit_period_sgadvanced=, explicit_period=off, period=1, dbl_ovrd_sgadvanced=, dbl_ovrd=off, use_behavioral_HDL_sgadvanced=, use_behavioral_HDL=off, use_rpm_sgadvanced=, use_rpm=off, xl_use_area_sgadvanced=, xl_use_area=off, xl_area=[0,0,0,0,0,0,0], xlcconfig=, has_advanced_control=0, sggui_pos=20,20,356,630, block_type=counter, block_version=8.2, sg_icon_stat=40,31,2,1,white,blue,0,eceade92, sg_mask_display=|, sg_list_contents=, sg_blockgui_xml=}
      mask sg_mask_display=|
      | fprintf('','COMMENT: begin icon graphics');
      | patch([0 40 40 0 ],[0 0 31 31 ],[0.77 0.82 0.91]);
      | patch([12 7 14 7 12 20 22 24 33 26 19 14 21 14 19 26 33 24 22 20 12 ],[3 8 15 22 27 27 25 27 27 20 27 22 15 8 3 10 3 3 5 3 3 ],[0.98 0.96 0.92]);
      | plot([0 0 40 40 0 ],[0 31 31 0 0 ]);
      | fprintf('','COMMENT: end icon graphics');
      | fprintf('','COMMENT: begin icon text');
      | color('black');port_label('input',1,'rst');
      | color('black');port_label('input',2,'en');
      | color('black');port_label('output',1,'out');
      | fprintf('','COMMENT: end icon text');
      mask prompts: infoedit ""; cnt_type_sgadvanced ""; cnt_type "Counter type"; cnt_to "Count to value"; operation_sgadvanced ""; operation "Count direction"; start_count "Initial value"; cnt_by_val "Step"; arith_type_sgadvanced ""; arith_type "Output type"; n_bits "Number of bits"; bin_pt "Binary point"; load_pin_sgadvanced ""; load_pin "Provide load port"; rst_sgadvanced ""; rst "Provide synchronous reset port"; en_sgadvanced ""; en "Provide enable port"; explicit_period_sgadvanced ""; explicit_period "Sample period source"; period "Explicit period"; dbl_ovrd_sgadvanced ""; dbl_ovrd "Override with doubles"; use_behavioral_HDL_sgadvanced ""; use_behavioral_HDL "Use behavioral HDL (otherwise use core)"; use_rpm_sgadvanced ""; use_rpm "Use pre-defined core placement information"; xl_use_area_sgadvanced ""; xl_use_area "Define FPGA area for resource estimation"; xl_area "FPGA area [slices, FFs, BRAMs, LUTs, IOBs, emb. mults, TBUFs]"; xlcconfig ""; has_advanced_control ""; sggui_pos ""; block_type ""; block_version ""; sg_icon_stat ""; sg_mask_display ""; sg_list_contents ""; sg_blockgui_xml ""
      mask help: Hardware notes: Free running counters are the least expensive in hardware. A count limited counter is implemented by combining a counter with a comparator.
      mask init: same as warplab_mimo_4x4/RSSI Clock Generator
      settings: CopyFcn=xlBlockMoveCallback(gcbh);  DeleteFcn=xlDestroyGui(gcbh);  ModelCloseFcn=xlDestroyGui(gcbh);  PreSaveFcn=xlBlockPreSaveCallback(gcbh);  PostSaveFcn=xlBlockPostSaveCallback(gcbh);  DestroyFcn=xlDestroyGui(gcbh);  OpenFcn=xlOpenGui(gcbh, 'counter_gui.xml', @counterenablement, -1)  CloseFcn=xlDestroyGui(gcbh);  MoveFcn=xlBlockMoveCallback(gcbh);
      mask Help: eval('xlWeb(xlhtmldoclink(''Counter''))');
      mask StyleString: edit,edit,popup(Free Running|Count Limited),edit,edit,popup(Up|Down|Up/Down),edit,edit,edit,popup(Signed  (2's comp)|Unsigned),edit,edit,edit,checkbox,edit,checkbox,edit,checkbox,edit,popup(on|off),edit,edit,checkbox,edit,checkbox,edit,checkbox,edit,checkbox,edit,edit,edit,edit,edit,edit,edit,edit,edit,edit
      mask Display:
      | fprintf('','COMMENT: begin icon graphics');
      | patch([0 40 40 0 ],[0 0 31 31 ],[0.77 0.82 0.91]);
      | patch([12 7 14 7 12 20 22 24 33 26 19 14 21 14 19 26 33 24 22 20 12 ],[3 8 15 22 27 27 25 27 27 20 27 22 15 8 3 10 3 3 5 3 3 ],[0.98 0.96 0.92]);
      | plot([0 0 40 40 0 ],[0 31 31 0 0 ]);
      | fprintf('','COMMENT: end icon graphics');
      | fprintf('','COMMENT: begin icon text');
      | color('black');port_label('input',1,'rst');
      | color('black');port_label('input',2,'en');
      | color('black');port_label('output',1,'out');
      | fprintf('','COMMENT: end icon text');
  debug_Capturing : S-Function  LoadFcn=xlBlockLoadCallback(gcbh);  FunctionName=sysgen  Parameters=ptable_  mask(Xilinx Gateway Out Block){infoedit=Gateway out block.  Converts Xilinx fixed point inputs into ouputs of type Simulink integer, double, or fixed point.<P><P>Hardware notes:  In hardware these blocks become top level output ports or are discarded, depending on how they are configured., hdl_port_sgadvanced=, hdl_port=on, timing_constraint_sgadvanced=, timing_constraint=None, locs_specified_sgadvanced=, locs_specified=off, LOCs={}, xl_use_area_sgadvanced=, xl_use_area=off, xl_area=[0,0,0,0,0,0,0], sginterface=, has_advanced_control=0, sggui_pos=-1,-1,-1,-1, block_type=gatewayout, block_version=8.2, sg_icon_stat=40,14,1,1,white,yellow,0,f0cec300, sg_mask_display=|, sg_list_contents=, sg_blockgui_xml=}
      mask sg_mask_display=|
      | fprintf('','COMMENT: begin icon graphics');
      | patch([0 40 40 0 ],[0 0 14 14 ],[0.95 0.93 0.65]);
      | patch([16 14 17 14 16 20 21 22 26 23 20 18 21 18 20 23 26 22 21 20 16 ],[2 4 7 10 12 12 11 12 12 9 12 10 7 4 2 5 2 2 3 2 2 ],[0.98 0.96 0.92]);
      | plot([0 0 40 40 0 ],[0 14 14 0 0 ]);
      | fprintf('','COMMENT: end icon graphics');
      | fprintf('','COMMENT: begin icon text');
      | color('black');port_label('input',1,' ');
      | color('black');port_label('output',1,'\fontsize{11pt}\bf Out ','texmode','on');
      | fprintf('','COMMENT: end icon text');
      mask prompts: infoedit ""; hdl_port_sgadvanced ""; hdl_port "Translate into output port"; timing_constraint_sgadvanced ""; timing_constraint "IOB timing constraint"; locs_specified_sgadvanced ""; locs_specified "Specify IOB location constraints"; LOCs "IOB pad locations (cell array {'MSB', ..., 'LSB'})"; xl_use_area_sgadvanced ""; xl_use_area "Define FPGA area for resource estimation"; xl_area "FPGA area [slices, FFs, BRAMs, LUTs, IOBs, emb. mults, TBUFs]"; sginterface ""; has_advanced_control ""; sggui_pos ""; block_type ""; block_version ""; sg_icon_stat ""; sg_mask_display ""; sg_list_contents ""; sg_blockgui_xml ""
      mask help:
      | Gateway out block.  Converts Xilinx fixed point inputs into ouputs of type Simulink integer, double, or fixed point.
      |
      | Hardware notes:  In hardware these blocks become top level output ports or are discarded, depending on how they are configured.
      mask init: same as warplab_mimo_4x4/RSSI_ADC_CLK
      settings: CopyFcn=xlBlockMoveCallback(gcbh);  DeleteFcn=xlDestroyGui(gcbh);  ModelCloseFcn=xlDestroyGui(gcbh);  PreSaveFcn=xlBlockPreSaveCallback(gcbh);  PostSaveFcn=xlBlockPostSaveCallback(gcbh);  DestroyFcn=xlDestroyGui(gcbh);  OpenFcn=xlOpenGui(gcbh, 'gatewayout_gui.xml', @gatewayoutenablement, -1)  CloseFcn=xlDestroyGui(gcbh);  MoveFcn=xlBlockMoveCallback(gcbh);
      mask Help: eval('xlWeb(xlhtmldoclink(''Gateway Out''))');
      mask StyleString: edit,edit,checkbox,edit,popup(None|Data Rate|Data Rate;  Set 'FAST' Attribute),edit,checkbox,edit,edit,checkbox,edit,edit,edit,edit,edit,edit,edit,edit,edit,edit
      mask Display:
      | fprintf('','COMMENT: begin icon graphics');
      | patch([0 40 40 0 ],[0 0 14 14 ],[0.95 0.93 0.65]);
      | patch([16 14 17 14 16 20 21 22 26 23 20 18 21 18 20 23 26 22 21 20 16 ],[2 4 7 10 12 12 11 12 12 9 12 10 7 4 2 5 2 2 3 2 2 ],[0.98 0.96 0.92]);
      | plot([0 0 40 40 0 ],[0 14 14 0 0 ]);
      | fprintf('','COMMENT: end icon graphics');
      | fprintf('','COMMENT: begin icon text');
      | color('black');port_label('input',1,' ');
      | color('black');port_label('output',1,'\fontsize{11pt}\bf Out ','texmode','on');
      | fprintf('','COMMENT: end icon text');
  debug_Transmitting : S-Function  LoadFcn=xlBlockLoadCallback(gcbh);  FunctionName=sysgen  Parameters=ptable_  mask(Xilinx Gateway Out Block){infoedit=Gateway out block.  Converts Xilinx fixed point inputs into ouputs of type Simulink integer, double, or fixed point.<P><P>Hardware notes:  In hardware these blocks become top level output ports or are discarded, depending on how they are configured., hdl_port_sgadvanced=, hdl_port=on, timing_constraint_sgadvanced=, timing_constraint=None, locs_specified_sgadvanced=, locs_specified=off, LOCs={}, xl_use_area_sgadvanced=, xl_use_area=off, xl_area=[0,0,0,0,0,0,0], sginterface=, has_advanced_control=0, sggui_pos=-1,-1,-1,-1, block_type=gatewayout, block_version=8.2, sg_icon_stat=40,14,1,1,white,yellow,0,f0cec300, sg_mask_display=|, sg_list_contents=, sg_blockgui_xml=}
      mask sg_mask_display=|
      | fprintf('','COMMENT: begin icon graphics');
      | patch([0 40 40 0 ],[0 0 14 14 ],[0.95 0.93 0.65]);
      | patch([16 14 17 14 16 20 21 22 26 23 20 18 21 18 20 23 26 22 21 20 16 ],[2 4 7 10 12 12 11 12 12 9 12 10 7 4 2 5 2 2 3 2 2 ],[0.98 0.96 0.92]);
      | plot([0 0 40 40 0 ],[0 14 14 0 0 ]);
      | fprintf('','COMMENT: end icon graphics');
      | fprintf('','COMMENT: begin icon text');
      | color('black');port_label('input',1,' ');
      | color('black');port_label('output',1,'\fontsize{11pt}\bf Out ','texmode','on');
      | fprintf('','COMMENT: end icon text');
      mask prompts: infoedit ""; hdl_port_sgadvanced ""; hdl_port "Translate into output port"; timing_constraint_sgadvanced ""; timing_constraint "IOB timing constraint"; locs_specified_sgadvanced ""; locs_specified "Specify IOB location constraints"; LOCs "IOB pad locations (cell array {'MSB', ..., 'LSB'})"; xl_use_area_sgadvanced ""; xl_use_area "Define FPGA area for resource estimation"; xl_area "FPGA area [slices, FFs, BRAMs, LUTs, IOBs, emb. mults, TBUFs]"; sginterface ""; has_advanced_control ""; sggui_pos ""; block_type ""; block_version ""; sg_icon_stat ""; sg_mask_display ""; sg_list_contents ""; sg_blockgui_xml ""
      mask help:
      | Gateway out block.  Converts Xilinx fixed point inputs into ouputs of type Simulink integer, double, or fixed point.
      |
      | Hardware notes:  In hardware these blocks become top level output ports or are discarded, depending on how they are configured.
      mask init: same as warplab_mimo_4x4/RSSI_ADC_CLK
      settings: CopyFcn=xlBlockMoveCallback(gcbh);  DeleteFcn=xlDestroyGui(gcbh);  ModelCloseFcn=xlDestroyGui(gcbh);  PreSaveFcn=xlBlockPreSaveCallback(gcbh);  PostSaveFcn=xlBlockPostSaveCallback(gcbh);  DestroyFcn=xlDestroyGui(gcbh);  OpenFcn=xlOpenGui(gcbh, 'gatewayout_gui.xml', @gatewayoutenablement, -1)  CloseFcn=xlDestroyGui(gcbh);  MoveFcn=xlBlockMoveCallback(gcbh);
      mask Help: eval('xlWeb(xlhtmldoclink(''Gateway Out''))');
      mask StyleString: edit,edit,checkbox,edit,popup(None|Data Rate|Data Rate;  Set 'FAST' Attribute),edit,checkbox,edit,edit,checkbox,edit,edit,edit,edit,edit,edit,edit,edit,edit,edit
      mask Display:
      | fprintf('','COMMENT: begin icon graphics');
      | patch([0 40 40 0 ],[0 0 14 14 ],[0.95 0.93 0.65]);
      | patch([16 14 17 14 16 20 21 22 26 23 20 18 21 18 20 23 26 22 21 20 16 ],[2 4 7 10 12 12 11 12 12 9 12 10 7 4 2 5 2 2 3 2 2 ],[0.98 0.96 0.92]);
      | plot([0 0 40 40 0 ],[0 14 14 0 0 ]);
      | fprintf('','COMMENT: end icon graphics');
      | fprintf('','COMMENT: begin icon text');
      | color('black');port_label('input',1,' ');
      | color('black');port_label('output',1,'\fontsize{11pt}\bf Out ','texmode','on');
      | fprintf('','COMMENT: end icon text');
  p_select : Subsystem  mask(pselect){C_BASE=0, C_HIGH=589823, C_OPB_AWIDTH=32, C_OPB_DWIDTH=32}
      mask prompts: C_BASE "Base Address"; C_HIGH "High Address"; C_OPB_AWIDTH "Address Bus Bit Width"; C_OPB_DWIDTH "Data Bus Bit Width"
      mask help: Address Decoding Logic
      mask init:
      | mdlGlobal = xlglobal(bdroot(gcbh));
      | if iskey(mdlGlobal,'mdlHandle')
      |   put(mdlGlobal,'opb_export_tool_v2_c_base', C_BASE);
      |   put(mdlGlobal,'opb_export_tool_v2_c_high', C_HIGH);
      |   put(mdlGlobal,'opb_export_tool_v2_c_opb_awidth', C_OPB_AWIDTH);
      |   put(mdlGlobal,'opb_export_tool_v2_c_opb_dwidth', C_OPB_DWIDTH);
      | end
  tag scope: ps=global
  wires:
  Posedge/1(Q) -> Mem_Control/1(Start)
  Pulse Generator/1 -> StartCapture/1
  Logical/1 -> Posedge/1(D)
  StartCapture/1 -> Logical/1
  Tx Addr Counter/1 -> Relational/1, Radio_1 Tx_Buffer/1(RdAddr), Radio_2 Tx_Buffer/1(RdAddr), Radio_3 Tx_Buffer/1(RdAddr), Radio_4 Tx_Buffer/1(RdAddr), Scope/7
  S-R_Latch/1(Q) -> Inverter/1, Tx Addr Counter/2, debug_Transmitting/1, Scope/6
  Relational/1 -> S-R_Latch/2(R)
  Inverter/1 -> Radio_1 Tx_Buffer/2(Rst), Tx Addr Counter/1, Radio_2 Tx_Buffer/2(Rst), Radio_3 Tx_Buffer/2(Rst), Radio_4 Tx_Buffer/2(Rst), Scope/5
  Radio_1_Inputs/1(Radio 1 I/Q) -> Radio_1 Rx_Buffers/1(I/Q)
  RSSI Clock Generator/1 -> RSSI_ADC_CLK/1
  Posedge1/1(Q) -> S-R_Latch/1(S)
  Radio_2_Inputs/1(Radio 2 I/Q) -> Radio_2 Rx_Buffers/1(I/Q)
  Radio_4_Inputs/1(Radio 4 I/Q) -> Radio_4 Rx_Buffers/1(I/Q)
  Radio_3_Inputs/1(Radio 3 I/Q) -> Radio_3 Rx_Buffers/1(I/Q)
  Pulse Generator1/1 -> StartTx/1
  StartTx/1 -> Logical1/1
  Logical1/1 -> Posedge1/1(D)
  Mem_Control/1(WrEn) -> CaptureDone/1(In1), debug_Capturing/1, Radio_2 Rx_Buffers/3(WE), Radio_1 Rx_Buffers/3(WE), Radio_3 Rx_Buffers/3(WE), Radio_4 Rx_Buffers/3(WE)
  Mem_Control/2(WrAddr) -> Radio_1 Rx_Buffers/2(Addr), Radio_2 Rx_Buffers/2(Addr), Radio_3 Rx_Buffers/2(Addr), Radio_4 Rx_Buffers/2(Addr)
  Radio_1 Tx_Buffer/1(Data) -> Radio_1_Outputs/1(32b), Scope/1
  Radio_2 Tx_Buffer/1(Data) -> Radio_2_Outputs/1(32b), Scope/2
  Radio_3 Tx_Buffer/1(Data) -> Radio_3_Outputs/1(32b), Scope/3
  Radio_4 Tx_Buffer/1(Data) -> Radio_4Outputs/1(32b), Scope/4
  [in_0] -> Mem_Control/3(CaptOffset)
  [in_1] -> Mem_Control/2(DoneReading)
  [in_2] -> Radio_2 Rx_Buffers/4(EN)
  [in_3] -> Radio_3 Rx_Buffers/4(EN)
  [in_4] -> Radio_4 Rx_Buffers/4(EN)
  [in_5] -> Logical/2
  [in_6] -> Logical1/2
  [in_7] -> Relational/2
  [in_8] -> Radio_1 Rx_Buffers/4(EN)
  [in_9] -> Radio_1 Tx_Buffer/3(En)
  [in_10] -> Radio_2 Tx_Buffer/3(En)
  [in_11] -> Radio_3 Tx_Buffer/3(En)
  [in_12] -> Radio_4 Tx_Buffer/3(En)
  [addr] -> p_select/1(addr)
  [a_valid] -> p_select/2(a_valid)
  p_select/1(ps) -> [ps]
  Mem_Control/3(WrAddr_zero) -> Radio_1 Rx_Buffers/5(Addr_zero), Radio_2 Rx_Buffers/5(Addr_zero), Radio_3 Rx_Buffers/5(Addr_zero), Radio_4 Rx_Buffers/5(Addr_zero)
